simulink model "simTP2_2023a"  (R2023a)
settings: Solver=ode4  StartTime=0.0  StopTime=10  FixedStep=1e-5  RelTol=1e-7
values from neighbouring files (symbols this model uses):
  dy0 = 0    [scriptTP2.m]
  g = 9.8    [scriptTP2.m]
  K = 0.0005    [scriptTP2.m]
  m = 0.1    [scriptTP2.m]
  y0 = 0.01    [scriptTP2.m]
settings Model: Creator=yariba  LastModifiedBy=yariba
settings ModelReferenceCC: EnableRefExpFcnMdlSchedulingChecks=on

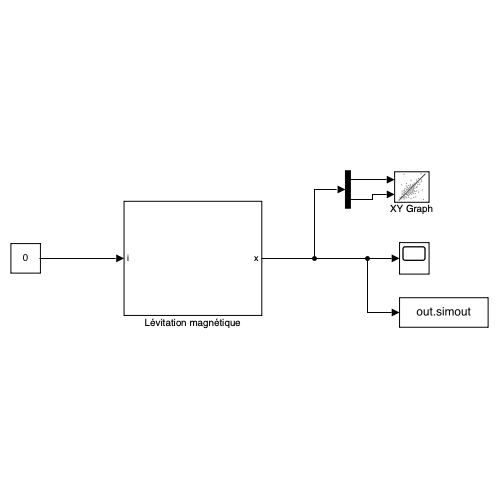
[thumbnail: Simulink's stored preview of the top-level diagram]
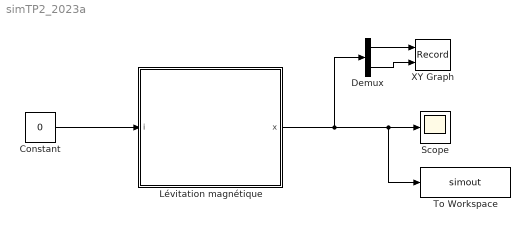
== system simTP2_2023a ==
  Constant : Constant  Value=0
  Demux : Demux  Outputs=2
  Lévitation magnétique : Subsystem
  Scope : Scope
  To Workspace : ToWorkspace  VariableName=simout  SaveFormat=Timeseries  SampleTime=-1
  XY Graph : Record  FileSettingsInternal="{\"entries\":[{\"content\":{\"excelSettings\":{\"content\":{},\"type\":\"Streamout.ExcelSettings\"}},\"type\":\"Streamout.FileSettingStorage\",\"uuid\":\"\"}],\"packageUris\":[\"http:\\/\\/schema.mathworks.com\\/mf0\\/streamout_blocks\\/R2020a\"],\"version\":\"1.0\"}"  Layout=[1 1]  SignalsInternal="{\"entries\":[{\"content\":{\"signals\":[{\"content\":{\"blockPath\":[],\"dimensions\":[1],\"domain\":\"\",\"lineColor\":\"#a2142f\",\"plots\":[ 1 ],\"port\":1,\"signalID\":1,\"signalName\":\"Demux:1\"},\"type\":\"RecordBlkView.Signal\",\"uuid\":\"\"},{\"content\":{\"blockPath\":[],\"dimensions\":[1],\"domain\":\"\",\"lineColor\":\"#139fff\",\"plots\":[ 1 ],\"port\":2,\"signalID\":2,\"signalName\":\"Demux:2\"},\"type\":\"RecordBlkView.Signal\",\"uuid\":\"\"}]},\"type\":\"RecordBlkView.InputSignals\",\"uuid\":\"\"}],\"packageUris\":[\"http:\\/\\/schema.mathworks.com\\/mf0\\/streamout_blocks\\/R2020a\"],\"version\":\"1.0\"}"  VisualizationBindings="{\"xyplotplugin\":{\"info\":[{\"series\":[{\"bindingParametersList\":[{\"parameter\":\"X-Axis\",\"signalID\":1,\"signalName\":\"Demux:1\"},{\"parameter\":\"Y-Axis\",\"signalID\":2,\"signalName\":\"Demux:2\"}],\"seriesID\":0}],\"subplotID\":1}]}}"  CompatibilityTag=XY
  wires:
  Lévitation magnétique/1(x) -> Demux/1, To Workspace/1, Scope/1
  Demux/1 -> XY Graph/1
  Demux/2 -> XY Graph/2
  Constant/1 -> Lévitation magnétique/1(i)

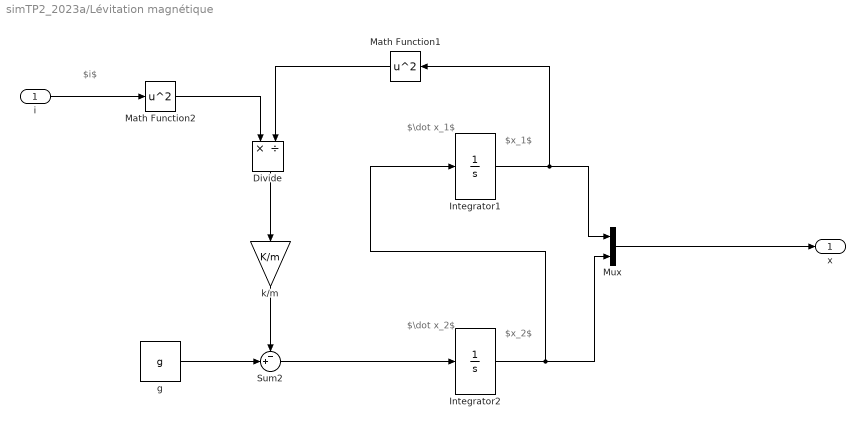
== system simTP2_2023a/Lévitation magnétique ==
  note: $x_1$
  note: $x_2$
  note: $\dot x_1$
  note: $\dot x_2$
  note: $i$
  i : Inport
  Divide : Product  Inputs=*/
  Integrator1 : Integrator  InitialCondition=y0
  Integrator2 : Integrator  InitialCondition=dy0
  Math Function1 : Math  Operator=square
  Math Function2 : Math  Operator=square
  Mux : Mux  Inputs=2
  Sum2 : Sum  Inputs=-+|
  g : Constant  Value=g
  k/m : Gain  Gain=K/m
  x : Outport
  wires:
  Integrator2/1 -> Integrator1/1, Mux/2
  Divide/1 -> k/m/1
  Mux/1 -> x/1
  Integrator1/1 -> Math Function1/1, Mux/1
  k/m/1 -> Sum2/1
  Sum2/1 -> Integrator2/1
  g/1 -> Sum2/2
  i/1 -> Math Function2/1
  Math Function1/1 -> Divide/2
  Math Function2/1 -> Divide/1
